simulink model "lab10q1_a"  (Simulink 7.1)
settings: Solver=ode45  StartTime=0.0  StopTime=0.2  RelTol=1e-3
InitFcn:
  | A = [1 1 0;-12 0 1;20 0 0]
  | 
  | B = [0;1;1]
  | 
  | C = [21 -1 1;1 0 0 ;0 1 0;0 0 1]
  | 
  | D=[0; 0; 0; 0]
settings Model: Creator=ALUNO  LastModifiedBy=ALUNO
settings DebuggingCC: SaveWithParameterizedLinksMsg=none

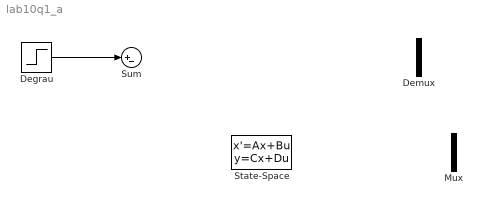
== system lab10q1_a ==
  Degrau : Step  Time=0  SampleTime=0
  Demux : Demux
  Mux : Mux  Inputs=2
  State-Space : StateSpace  A=A  B=B  C=C  D=D
  Sum : Sum  Inputs=|+-  OutDataType=sfix(16)  OutScaling=2^0
  wires:
  Degrau/1 -> Sum/1
